simulink model "mrefrobotarm_modified_previous_y_previous_u_previous_ref_pert"  (R2018b)
settings: Solver=FixedStepAuto  StartTime=0.0  StopTime=10  RelTol=1e-3  AbsTol=1e-6
undefined symbols (not defined in the file or in its folder): cc, options
libraries: neural x714, simulink x1
(part 14 of 26)

== system mrefrobotarm_modified_previous_y_previous_u_previous_ref_pert/no_ss_error/Layer 3/LW{3,2} ==
  "ad{3,2}" : Inport  PortDimensions=10
      mask Display: e = 0.06;c1 = [120 230 180]/255;c2 = ([120 230 180]+0)/(256+128);c3 = ([120 230 180]+128)/(256+128);patch([0 1 1 0],[0 0 1 1],c1);patch([0 1 1 1-e 1-e 0+e],[0 0 1 1-e 0+e 0+e],c2);patch([0 0 1 1-e 0+e 0+e],[0 1 1 1-e 1-e 0+e],c3);plot([0 1 1 0 0],[0 0 1 1 0]);
  "IW{3,2}(1,:)'" : Constant  Value=[-1.1742149213841346355735595352598465979099273681640625;-0.36956930765582274300840026626246981322765350341796875;-0.020974811427770558014405111180167295970022678375244140625;-0.1621617407977070934865793105927878059446811676025390625;-1.0555440515423846203901803164626471698284149169921875;0.9397318128967075967494793076184578239917755126953125;1.108386888893071908768206412787549197673797607421875;-1.6860005455705617816164476607809774577617645263671875;0.39441695259544518048500094664632342755794525146484375;0.311368724958305309602479837849386967718601226806640625]
      mask Display: e = 0.06;c1 = [120 150 230]/255;c2 = ([120 150 230]+0)/383;c3 = ([120 150 230]+128)/383;patch([0 1 1 0],[0 0 1 1],c1);patch([0 1 1 1-e 1-e 0+e],[0 0 1 1-e 0+e 0+e],c2);patch([0 0 1 1-e 0+e 0+e],[0 1 1 1-e 1-e 0+e],c3);plot([0 1 1 0 0],[0 0 1 1 0]);disp('weights');
  "IW{3,2}(10,:)'" : Constant  Value=[1.2868963402164153020379444569698534905910491943359375;1.0043335498955787699060238082893192768096923828125;0.357778577002095532488823437233804725110530853271484375;0.125142367753036942712441259573097340762615203857421875;0.329491920370458657441048444525222294032573699951171875;0.3719554364254389344779383463901467621326446533203125;0.094035472804396447177310847109765745699405670166015625;-1.5356693414710511635945522357360459864139556884765625;-0.234492704566690746137425094275386072695255279541015625;0.76033474886525265201697720840456895530223846435546875]
      mask Display: e = 0.06;c1 = [120 150 230]/255;c2 = ([120 150 230]+0)/383;c3 = ([120 150 230]+128)/383;patch([0 1 1 0],[0 0 1 1],c1);patch([0 1 1 1-e 1-e 0+e],[0 0 1 1-e 0+e 0+e],c2);patch([0 0 1 1-e 0+e 0+e],[0 1 1 1-e 1-e 0+e],c3);plot([0 1 1 0 0],[0 0 1 1 0]);disp('weights');
  "IW{3,2}(2,:)'" : Constant  Value=[-0.79821657120366451554360764930606819689273834228515625;-0.3531049846577680728643144902889616787433624267578125;-0.07096205186676474152562832387047819793224334716796875;1.0162264331966504027349174066330306231975555419921875;-0.04359937457296637897119495619335793890058994293212890625;-0.65589298183328781366441262434818781912326812744140625;-1.0034240677702126465220544559997506439685821533203125;-0.178302261212416823799031817543436773121356964111328125;0.26934055472063522795878043325501494109630584716796875;0.7890398483409157837087377629359252750873565673828125]
      mask Display: e = 0.06;c1 = [120 150 230]/255;c2 = ([120 150 230]+0)/383;c3 = ([120 150 230]+128)/383;patch([0 1 1 0],[0 0 1 1],c1);patch([0 1 1 1-e 1-e 0+e],[0 0 1 1-e 0+e 0+e],c2);patch([0 0 1 1-e 0+e 0+e],[0 1 1 1-e 1-e 0+e],c3);plot([0 1 1 0 0],[0 0 1 1 0]);disp('weights');
  "IW{3,2}(3,:)'" : Constant  Value=[0.34998478961192713843075807744753547012805938720703125;0.66241428248508438247910135032725520431995391845703125;0.1149456925372841775701004962684237398207187652587890625;-0.34497320121806829273936045865411870181560516357421875;-1.151869423380677659451976069249212741851806640625;-0.2339138016921568363759575959193171001970767974853515625;-0.494599686326340937103651640427415259182453155517578125;0.149782276593690977239958783684414811432361602783203125;0.30087508159218778747145961460773833096027374267578125;-1.0897169507045614267326527624391019344329833984375]
      mask Display: e = 0.06;c1 = [120 150 230]/255;c2 = ([120 150 230]+0)/383;c3 = ([120 150 230]+128)/383;patch([0 1 1 0],[0 0 1 1],c1);patch([0 1 1 1-e 1-e 0+e],[0 0 1 1-e 0+e 0+e],c2);patch([0 0 1 1-e 0+e 0+e],[0 1 1 1-e 1-e 0+e],c3);plot([0 1 1 0 0],[0 0 1 1 0]);disp('weights');
  "IW{3,2}(4,:)'" : Constant  Value=[-0.06940107506443075890967264740538666956126689910888671875;0.06031549876058779624532490970523213036358356475830078125;-0.258147786648753874150230558370822109282016754150390625;-0.0329451661351574387470719784687389619648456573486328125;0.93910292630476110975479286935296840965747833251953125;0.89089233434477754780544955792720429599285125732421875;-0.560766298108745786521467380225658416748046875;-0.72585852285035645792277136933989822864532470703125;0.674225279114710307482027928926981985569000244140625;0.1249268934935323371870907749325851909816265106201171875]
      mask Display: e = 0.06;c1 = [120 150 230]/255;c2 = ([120 150 230]+0)/383;c3 = ([120 150 230]+128)/383;patch([0 1 1 0],[0 0 1 1],c1);patch([0 1 1 1-e 1-e 0+e],[0 0 1 1-e 0+e 0+e],c2);patch([0 0 1 1-e 0+e 0+e],[0 1 1 1-e 1-e 0+e],c3);plot([0 1 1 0 0],[0 0 1 1 0]);disp('weights');
  "IW{3,2}(5,:)'" : Constant  Value=[1.0319694087142163851922305184416472911834716796875;-0.6356320185586259441379297641105949878692626953125;0.627606968594268010974701610393822193145751953125;-0.60009465064882083762398679027683101594448089599609375;0.36085902571910588587655865921988151967525482177734375;0.0166213576772036956963329856762356939725577831268310546875;0.68217943372506295585111502077779732644557952880859375;-0.260281007332698488543343273704522289335727691650390625;0.4773504187563932799065469225752167403697967529296875;-0.246983657567856285108831571051268838346004486083984375]
      mask Display: e = 0.06;c1 = [120 150 230]/255;c2 = ([120 150 230]+0)/383;c3 = ([120 150 230]+128)/383;patch([0 1 1 0],[0 0 1 1],c1);patch([0 1 1 1-e 1-e 0+e],[0 0 1 1-e 0+e 0+e],c2);patch([0 0 1 1-e 0+e 0+e],[0 1 1 1-e 1-e 0+e],c3);plot([0 1 1 0 0],[0 0 1 1 0]);disp('weights');
  "IW{3,2}(6,:)'" : Constant  Value=[0.59600639630389962153600436067790724337100982666015625;-0.6219517438347332838333159088506363332271575927734375;-0.28957206042188088357391961835674010217189788818359375;-0.6317708261151226967200500439503230154514312744140625;0.7916489865234155320905529151787050068378448486328125;1.1118173714307049149141448651789687573909759521484375;0.95397976829716701896444419617182575166225433349609375;0.264598423771943369597892115052673034369945526123046875;0.36001495974812003364462498211651109158992767333984375;0.43069856328655531374494103147299028933048248291015625]
      mask Display: e = 0.06;c1 = [120 150 230]/255;c2 = ([120 150 230]+0)/383;c3 = ([120 150 230]+128)/383;patch([0 1 1 0],[0 0 1 1],c1);patch([0 1 1 1-e 1-e 0+e],[0 0 1 1-e 0+e 0+e],c2);patch([0 0 1 1-e 0+e 0+e],[0 1 1 1-e 1-e 0+e],c3);plot([0 1 1 0 0],[0 0 1 1 0]);disp('weights');
  "IW{3,2}(7,:)'" : Constant  Value=[0.8347467852459591330926969021675176918506622314453125;0.64027222919503190556866911720135249197483062744140625;0.51949179774282805421847797333612106740474700927734375;0.330143188575668988793410107973613776266574859619140625;1.1088920656695460120744201049092225730419158935546875;-0.85106155681901174414605293350177817046642303466796875;-0.85451872016597718584307585842907428741455078125;-0.459549904446422186055087877321057021617889404296875;0.282431179270222931787515108226216398179531097412109375;-0.37750346721447958220352347780135460197925567626953125]
      mask Display: e = 0.06;c1 = [120 150 230]/255;c2 = ([120 150 230]+0)/383;c3 = ([120 150 230]+128)/383;patch([0 1 1 0],[0 0 1 1],c1);patch([0 1 1 1-e 1-e 0+e],[0 0 1 1-e 0+e 0+e],c2);patch([0 0 1 1-e 0+e 0+e],[0 1 1 1-e 1-e 0+e],c3);plot([0 1 1 0 0],[0 0 1 1 0]);disp('weights');
  "IW{3,2}(8,:)'" : Constant  Value=[0.34325135738398848683772257572854869067668914794921875;-1.01090554861465253821961596258915960788726806640625;1.302095617056524989862964503117837011814117431640625;-1.019798546469042666018367526703514158725738525390625;-1.9669407327809864671763762089540250599384307861328125;0.2982089316163587522368061399902217090129852294921875;0.04332335823831089116620063350637792609632015228271484375;-0.074115637045339133326393721290514804422855377197265625;0.54303975452732922146736882496043108403682708740234375;-0.1028235277364488720053259385167621076107025146484375]
      mask Display: e = 0.06;c1 = [120 150 230]/255;c2 = ([120 150 230]+0)/383;c3 = ([120 150 230]+128)/383;patch([0 1 1 0],[0 0 1 1],c1);patch([0 1 1 1-e 1-e 0+e],[0 0 1 1-e 0+e 0+e],c2);patch([0 0 1 1-e 0+e 0+e],[0 1 1 1-e 1-e 0+e],c3);plot([0 1 1 0 0],[0 0 1 1 0]);disp('weights');
  "IW{3,2}(9,:)'" : Constant  Value=[-0.2519934093643081407520867287530563771724700927734375;0.89673409560586414546179412354831583797931671142578125;-0.3290727524169818618560157119645737111568450927734375;-0.78288240927482222186739591052173636853694915771484375;0.357415489622151583137821262425859458744525909423828125;-0.0396763127742645327344916950096376240253448486328125;0.26571572727522230206176345745916478335857391357421875;0.65064151536380887552724061606568284332752227783203125;-0.2531486350804550422566308043315075337886810302734375;-0.375085198445921974563788126033614389598369598388671875]
      mask Display: e = 0.06;c1 = [120 150 230]/255;c2 = ([120 150 230]+0)/383;c3 = ([120 150 230]+128)/383;patch([0 1 1 0],[0 0 1 1],c1);patch([0 1 1 1-e 1-e 0+e],[0 0 1 1-e 0+e 0+e],c2);patch([0 0 1 1-e 0+e 0+e],[0 1 1 1-e 1-e 0+e],c3);plot([0 1 1 0 0],[0 0 1 1 0]);disp('weights');
  Mux : Mux  Inputs=10
      mask Display: e = 0.06;c1 = [120 150 230]/255;c2 = ([120 150 230]+0)/383;c3 = ([120 150 230]+128)/383;patch([0 1 1 0],[0 0 1 1],c1);patch([0 1 1 1-e 1-e 0+e],[0 0 1 1-e 0+e 0+e],c2);patch([0 0 1 1-e 0+e 0+e],[0 1 1 1-e 1-e 0+e],c3);plot([0 1 1 0 0],[0 0 1 1 0]);disp('Mux');
  dotprod{1..10} (10 alike) : neural/Weight Functions/dotprod
  "lz{3,2}" : Outport
      mask Display: e = 0.06;c1 = [120 230 180]/255;c2 = ([120 230 180]+0)/(256+128);c3 = ([120 230 180]+128)/(256+128);patch([0 1 1 0],[0 0 1 1],c1);patch([0 1 1 1-e 1-e 0+e],[0 0 1 1-e 0+e 0+e],c2);patch([0 0 1 1-e 0+e 0+e],[0 1 1 1-e 1-e 0+e],c3);plot([0 1 1 0 0],[0 0 1 1 0]);
  wires:
  "IW{3,2}(1,:)'"/1 -> dotprod1/1
  "ad{3,2}"/1 -> dotprod1/2, dotprod2/2, dotprod3/2, dotprod4/2, dotprod5/2, dotprod6/2, dotprod7/2, dotprod8/2, dotprod9/2, dotprod10/2
  dotprod1/1 -> Mux/1
  "IW{3,2}(2,:)'"/1 -> dotprod2/1
  dotprod2/1 -> Mux/2
  "IW{3,2}(3,:)'"/1 -> dotprod3/1
  dotprod3/1 -> Mux/3
  "IW{3,2}(4,:)'"/1 -> dotprod4/1
  dotprod4/1 -> Mux/4
  "IW{3,2}(5,:)'"/1 -> dotprod5/1
  dotprod5/1 -> Mux/5
  "IW{3,2}(6,:)'"/1 -> dotprod6/1
  dotprod6/1 -> Mux/6
  "IW{3,2}(7,:)'"/1 -> dotprod7/1
  dotprod7/1 -> Mux/7
  "IW{3,2}(8,:)'"/1 -> dotprod8/1
  dotprod8/1 -> Mux/8
  "IW{3,2}(9,:)'"/1 -> dotprod9/1
  dotprod9/1 -> Mux/9
  "IW{3,2}(10,:)'"/1 -> dotprod10/1
  dotprod10/1 -> Mux/10
  Mux/1 -> "lz{3,2}"/1

== system mrefrobotarm_modified_previous_y_previous_u_previous_ref_pert/no_ss_error/Layer 4/Delays 1 ==
  "p{4}" : Inport  PortDimensions=10
      mask Display: e = 0.06;c1 = [120 230 180]/255;c2 = ([120 230 180]+0)/(256+128);c3 = ([120 230 180]+128)/(256+128);patch([0 1 1 0],[0 0 1 1],c1);patch([0 1 1 1-e 1-e 0+e],[0 0 1 1-e 0+e 0+e],c2);patch([0 0 1 1-e 0+e 0+e],[0 1 1 1-e 1-e 0+e],c3);plot([0 1 1 0 0],[0 0 1 1 0]);
  mux : Mux  Inputs=1
      mask Display: e = 0.06;c1 = [120 150 230]/255;c2 = ([120 150 230]+0)/383;c3 = ([120 150 230]+128)/383;patch([0 1 1 0],[0 0 1 1],c1);patch([0 1 1 1-e 1-e 0+e],[0 0 1 1-e 0+e 0+e],c2);patch([0 0 1 1-e 0+e 0+e],[0 1 1 1-e 1-e 0+e],c3);plot([0 1 1 0 0],[0 0 1 1 0]);disp('Mux')
  "pd{4,3}" : Outport
      mask Display: e = 0.06;c1 = [120 230 180]/255;c2 = ([120 230 180]+0)/(256+128);c3 = ([120 230 180]+128)/(256+128);patch([0 1 1 0],[0 0 1 1],c1);patch([0 1 1 1-e 1-e 0+e],[0 0 1 1-e 0+e 0+e],c2);patch([0 0 1 1-e 0+e 0+e],[0 1 1 1-e 1-e 0+e],c3);plot([0 1 1 0 0],[0 0 1 1 0]);
  wires:
  "p{4}"/1 -> mux/1
  mux/1 -> "pd{4,3}"/1

== system mrefrobotarm_modified_previous_y_previous_u_previous_ref_pert/no_ss_error/Layer 4/LW{4,3} ==
  "ad{4,3}" : Inport  PortDimensions=10
      mask Display: e = 0.06;c1 = [120 230 180]/255;c2 = ([120 230 180]+0)/(256+128);c3 = ([120 230 180]+128)/(256+128);patch([0 1 1 0],[0 0 1 1],c1);patch([0 1 1 1-e 1-e 0+e],[0 0 1 1-e 0+e 0+e],c2);patch([0 0 1 1-e 0+e 0+e],[0 1 1 1-e 1-e 0+e],c3);plot([0 1 1 0 0],[0 0 1 1 0]);
  "IW{4,3}(1,:)'" : Constant  Value=[-0.2284255511763977342098996814456768333911895751953125;0.326359030917801773430397815900505520403385162353515625;0.7413839295182060862288153657573275268077850341796875;-0.359416929133310414368196461509796790778636932373046875;0.359071647237452495904364013767917640507221221923828125;-0.1211637014833257530721510875082458369433879852294921875;0.128617773868923757074611557982279919087886810302734375;-0.890162829817878975546818764996714890003204345703125;0.957733879752896921644378380733542144298553466796875;1.054540145396258399301814279169775545597076416015625]
      mask Display: e = 0.06;c1 = [120 150 230]/255;c2 = ([120 150 230]+0)/383;c3 = ([120 150 230]+128)/383;patch([0 1 1 0],[0 0 1 1],c1);patch([0 1 1 1-e 1-e 0+e],[0 0 1 1-e 0+e 0+e],c2);patch([0 0 1 1-e 0+e 0+e],[0 1 1 1-e 1-e 0+e],c3);plot([0 1 1 0 0],[0 0 1 1 0]);disp('weights');
  Mux : Mux  Inputs=1
      mask Display: e = 0.06;c1 = [120 150 230]/255;c2 = ([120 150 230]+0)/383;c3 = ([120 150 230]+128)/383;patch([0 1 1 0],[0 0 1 1],c1);patch([0 1 1 1-e 1-e 0+e],[0 0 1 1-e 0+e 0+e],c2);patch([0 0 1 1-e 0+e 0+e],[0 1 1 1-e 1-e 0+e],c3);plot([0 1 1 0 0],[0 0 1 1 0]);disp('Mux');
  dotprod1 : neural/Weight Functions/dotprod
  "lz{4,3}" : Outport
      mask Display: e = 0.06;c1 = [120 230 180]/255;c2 = ([120 230 180]+0)/(256+128);c3 = ([120 230 180]+128)/(256+128);patch([0 1 1 0],[0 0 1 1],c1);patch([0 1 1 1-e 1-e 0+e],[0 0 1 1-e 0+e 0+e],c2);patch([0 0 1 1-e 0+e 0+e],[0 1 1 1-e 1-e 0+e],c3);plot([0 1 1 0 0],[0 0 1 1 0]);
  wires:
  "IW{4,3}(1,:)'"/1 -> dotprod1/1
  "ad{4,3}"/1 -> dotprod1/2
  dotprod1/1 -> Mux/1
  Mux/1 -> "lz{4,3}"/1

== system mrefrobotarm_modified_previous_y_previous_u_previous_ref_pert/sd=0.001/Layer 1/Delays 1 ==
  "p{1}" : Inport  PortDimensions=10
      mask Display: e = 0.06;c1 = [120 230 180]/255;c2 = ([120 230 180]+0)/(256+128);c3 = ([120 230 180]+128)/(256+128);patch([0 1 1 0],[0 0 1 1],c1);patch([0 1 1 1-e 1-e 0+e],[0 0 1 1-e 0+e 0+e],c2);patch([0 0 1 1-e 0+e 0+e],[0 1 1 1-e 1-e 0+e],c3);plot([0 1 1 0 0],[0 0 1 1 0]);
  mux : Mux  Inputs=1
      mask Display: e = 0.06;c1 = [120 150 230]/255;c2 = ([120 150 230]+0)/383;c3 = ([120 150 230]+128)/383;patch([0 1 1 0],[0 0 1 1],c1);patch([0 1 1 1-e 1-e 0+e],[0 0 1 1-e 0+e 0+e],c2);patch([0 0 1 1-e 0+e 0+e],[0 1 1 1-e 1-e 0+e],c3);plot([0 1 1 0 0],[0 0 1 1 0]);disp('Mux')
  "pd{1,1}" : Outport
      mask Display: e = 0.06;c1 = [120 230 180]/255;c2 = ([120 230 180]+0)/(256+128);c3 = ([120 230 180]+128)/(256+128);patch([0 1 1 0],[0 0 1 1],c1);patch([0 1 1 1-e 1-e 0+e],[0 0 1 1-e 0+e 0+e],c2);patch([0 0 1 1-e 0+e 0+e],[0 1 1 1-e 1-e 0+e],c3);plot([0 1 1 0 0],[0 0 1 1 0]);
  wires:
  "p{1}"/1 -> mux/1
  mux/1 -> "pd{1,1}"/1

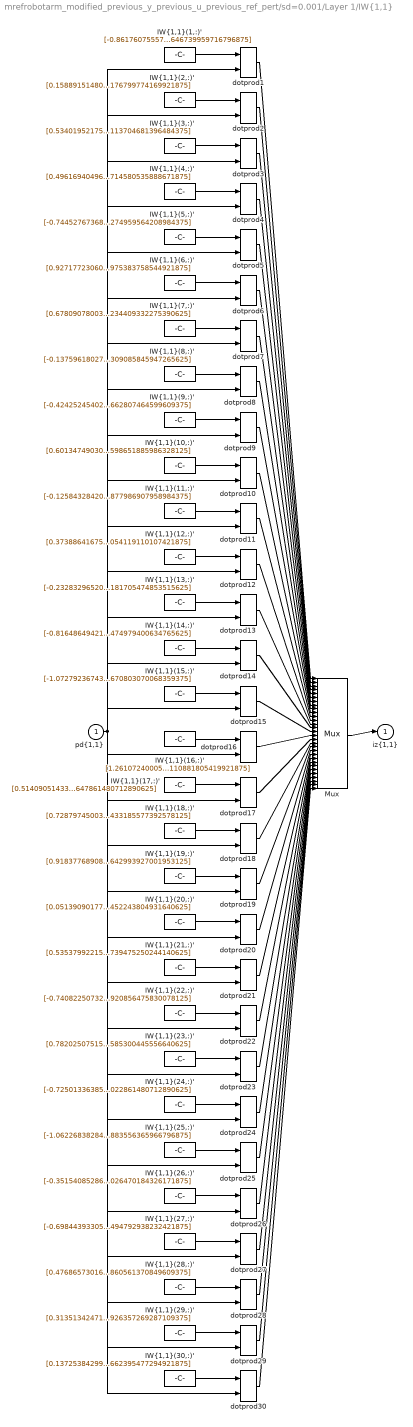
== system mrefrobotarm_modified_previous_y_previous_u_previous_ref_pert/sd=0.001/Layer 1/IW{1,1} ==
  "pd{1,1}" : Inport  PortDimensions=10
      mask Display: e = 0.06;c1 = [120 230 180]/255;c2 = ([120 230 180]+0)/(256+128);c3 = ([120 230 180]+128)/(256+128);patch([0 1 1 0],[0 0 1 1],c1);patch([0 1 1 1-e 1-e 0+e],[0 0 1 1-e 0+e 0+e],c2);patch([0 0 1 1-e 0+e 0+e],[0 1 1 1-e 1-e 0+e],c3);plot([0 1 1 0 0],[0 0 1 1 0]);
  "IW{1,1}(1,:)'" : Constant  Value=[-0.86176075557723141873367467269417829811573028564453125;0.004071028969782842545088730190627757110632956027984619140625;0.9276173767568607342326458820025436580181121826171875;-0.7967440168978880965511280010105110704898834228515625;0.1354921212385334639005662893396220169961452484130859375;0.8229380829797723340135462422040291130542755126953125;-0.89325111752537622589187549237976782023906707763671875;-0.040687801222941966106105837752693332731723785400390625;0.1879890646825829458865797505495720542967319488525390625;0.66378054058433366702018929572659544646739959716796875]
      mask Display: e = 0.06;c1 = [120 150 230]/255;c2 = ([120 150 230]+0)/383;c3 = ([120 150 230]+128)/383;patch([0 1 1 0],[0 0 1 1],c1);patch([0 1 1 1-e 1-e 0+e],[0 0 1 1-e 0+e 0+e],c2);patch([0 0 1 1-e 0+e 0+e],[0 1 1 1-e 1-e 0+e],c3);plot([0 1 1 0 0],[0 0 1 1 0]);disp('Weights');
  "IW{1,1}(10,:)'" : Constant  Value=[0.6013474903013322769851356497383676469326019287109375;0.2357213474255306639992824102591839618980884552001953125;0.0312087080959108920108491247447091154754161834716796875;-0.72882097215190777550475331736379303038120269775390625;0.27025423916619695230423303655697964131832122802734375;-0.15361402603164375779698502810788340866565704345703125;0.78092852510657195796994756165076978504657745361328125;1.1338252142460525373479640620644204318523406982421875;0.8835122077703960741246191901154816150665283203125;-0.57041135401077724953466940860380418598651885986328125]
      mask Display: e = 0.06;c1 = [120 150 230]/255;c2 = ([120 150 230]+0)/383;c3 = ([120 150 230]+128)/383;patch([0 1 1 0],[0 0 1 1],c1);patch([0 1 1 1-e 1-e 0+e],[0 0 1 1-e 0+e 0+e],c2);patch([0 0 1 1-e 0+e 0+e],[0 1 1 1-e 1-e 0+e],c3);plot([0 1 1 0 0],[0 0 1 1 0]);disp('Weights');
  "IW{1,1}(11,:)'" : Constant  Value=[-0.1258432842075885293997572489388403482735157012939453125;-0.95290940317177341700727311035734601318836212158203125;0.3798642085459082995413382377591915428638458251953125;-0.47392543300202205625026863344828598201274871826171875;0.284850629948106226496662429781281389296054840087890625;-0.37713871544512567179907591707888059318065643310546875;0.52725521709343647902556995177292264997959136962890625;0.6632129839156402084654473583213984966278076171875;1.1084132506835449039073182575521059334278106689453125;-0.42571958046212843296274286331026814877986907958984375]
      mask Display: e = 0.06;c1 = [120 150 230]/255;c2 = ([120 150 230]+0)/383;c3 = ([120 150 230]+128)/383;patch([0 1 1 0],[0 0 1 1],c1);patch([0 1 1 1-e 1-e 0+e],[0 0 1 1-e 0+e 0+e],c2);patch([0 0 1 1-e 0+e 0+e],[0 1 1 1-e 1-e 0+e],c3);plot([0 1 1 0 0],[0 0 1 1 0]);disp('Weights');
  "IW{1,1}(12,:)'" : Constant  Value=[0.373886416754146966301419752198853529989719390869140625;-0.53407118968250644197581777916639111936092376708984375;-0.974687317709341360938424259074963629245758056640625;-0.81026545963209606338040202899719588458538055419921875;1.2545756075142449059711680092732422053813934326171875;-1.403611791985415191419406255590729415416717529296875;1.0287428745390150286453945227549411356449127197265625;0.73290349012389544025580789821106009185314178466796875;0.11950116559000185934014126587499049492180347442626953125;-0.6581982943801925056703794325585477054119110107421875]
      mask Display: e = 0.06;c1 = [120 150 230]/255;c2 = ([120 150 230]+0)/383;c3 = ([120 150 230]+128)/383;patch([0 1 1 0],[0 0 1 1],c1);patch([0 1 1 1-e 1-e 0+e],[0 0 1 1-e 0+e 0+e],c2);patch([0 0 1 1-e 0+e 0+e],[0 1 1 1-e 1-e 0+e],c3);plot([0 1 1 0 0],[0 0 1 1 0]);disp('Weights');
  "IW{1,1}(13,:)'" : Constant  Value=[-0.2328329652087623158340790041620493866503238677978515625;0.25214791019473847821785739142796956002712249755859375;-0.857616619290316517520977868116460740566253662109375;0.1597045671382539833160763009800575673580169677734375;-0.89199095776851045069832935041631571948528289794921875;-0.40844745584091957102401693191495724022388458251953125;0.416911726643029556527153545175679028034210205078125;0.44604718664590847776452164907823316752910614013671875;-1.0838179239725198588217836004332639276981353759765625;-1.4845463738733233327593552530743181705474853515625]
      mask Display: e = 0.06;c1 = [120 150 230]/255;c2 = ([120 150 230]+0)/383;c3 = ([120 150 230]+128)/383;patch([0 1 1 0],[0 0 1 1],c1);patch([0 1 1 1-e 1-e 0+e],[0 0 1 1-e 0+e 0+e],c2);patch([0 0 1 1-e 0+e 0+e],[0 1 1 1-e 1-e 0+e],c3);plot([0 1 1 0 0],[0 0 1 1 0]);disp('Weights');
  "IW{1,1}(14,:)'" : Constant  Value=[-0.81648649421498709077837929726229049265384674072265625;-0.1711459426988634902055963493694434873759746551513671875;0.3309884131682216956704678523237816989421844482421875;0.5470694340943669242705027500051073729991912841796875;0.648293249569385832131729330285452306270599365234375;-0.8610077775310236436467903331504203379154205322265625;0.036703737521726009784828193005523644387722015380859375;-0.445491607745406081875216841581277549266815185546875;0.75751953895534140936973699353984557092189788818359375;0.067524437334262776833071484361425973474979400634765625]
      mask Display: e = 0.06;c1 = [120 150 230]/255;c2 = ([120 150 230]+0)/383;c3 = ([120 150 230]+128)/383;patch([0 1 1 0],[0 0 1 1],c1);patch([0 1 1 1-e 1-e 0+e],[0 0 1 1-e 0+e 0+e],c2);patch([0 0 1 1-e 0+e 0+e],[0 1 1 1-e 1-e 0+e],c3);plot([0 1 1 0 0],[0 0 1 1 0]);disp('Weights');
  "IW{1,1}(15,:)'" : Constant  Value=[-1.07279236743805572729115738184191286563873291015625;-0.22077776363054368857774534262716770172119140625;-1.1441750592332462499456369187100790441036224365234375;-0.0243684922136943975246037297210932592861354351043701171875;0.6338152544858817183381916038342751562595367431640625;-0.3991749720177695248679583528428338468074798583984375;-0.033335841958008184671147233757437788881361484527587890625;-0.405257397821079445865422030692570842802524566650390625;0.5599912552127384035571822096244432032108306884765625;-0.91172899721163103148313666679314337670803070068359375]
      mask Display: e = 0.06;c1 = [120 150 230]/255;c2 = ([120 150 230]+0)/383;c3 = ([120 150 230]+128)/383;patch([0 1 1 0],[0 0 1 1],c1);patch([0 1 1 1-e 1-e 0+e],[0 0 1 1-e 0+e 0+e],c2);patch([0 0 1 1-e 0+e 0+e],[0 1 1 1-e 1-e 0+e],c3);plot([0 1 1 0 0],[0 0 1 1 0]);disp('Weights');
  "IW{1,1}(16,:)'" : Constant  Value=[1.261072400056214792840592053835280239582061767578125;-0.448328322608864626719338275506743229925632476806640625;0.2280649357326325343819917179644107818603515625;-0.31922125582217242278915136921568773686885833740234375;2.2790899227644043634199988446198403835296630859375;-0.74094992287071204106752020379644818603992462158203125;-0.06839834232064727348454624689111369661986827850341796875;-0.361411436047278156191708831102005206048488616943359375;-0.274032669218069013794547572615556418895721435546875;0.431462257503983870332575634165550582110881805419921875]
      mask Display: e = 0.06;c1 = [120 150 230]/255;c2 = ([120 150 230]+0)/383;c3 = ([120 150 230]+128)/383;patch([0 1 1 0],[0 0 1 1],c1);patch([0 1 1 1-e 1-e 0+e],[0 0 1 1-e 0+e 0+e],c2);patch([0 0 1 1-e 0+e 0+e],[0 1 1 1-e 1-e 0+e],c3);plot([0 1 1 0 0],[0 0 1 1 0]);disp('Weights');
  "IW{1,1}(17,:)'" : Constant  Value=[0.5140905143300018576013599158613942563533782958984375;-0.9116222129188285006051728487364016473293304443359375;-0.1962638231180134085196442583765019662678241729736328125;0.186268042418468227072736453919787891209125518798828125;-0.1420763900966267867520542722559184767305850982666015625;-0.019898823210212468470814428656012751162052154541015625;-0.650313148725484513335004521650262176990509033203125;-0.8810028290455473864994928590022027492523193359375;-0.41969576868875713149265038737212307751178741455078125;0.9138742157549766265134394416236318647861480712890625]
      mask Display: e = 0.06;c1 = [120 150 230]/255;c2 = ([120 150 230]+0)/383;c3 = ([120 150 230]+128)/383;patch([0 1 1 0],[0 0 1 1],c1);patch([0 1 1 1-e 1-e 0+e],[0 0 1 1-e 0+e 0+e],c2);patch([0 0 1 1-e 0+e 0+e],[0 1 1 1-e 1-e 0+e],c3);plot([0 1 1 0 0],[0 0 1 1 0]);disp('Weights');
  "IW{1,1}(18,:)'" : Constant  Value=[0.728797450031771543166314586414955556392669677734375;-1.1059143967640452377310111842234618961811065673828125;-0.2346485878811759573370210318898898549377918243408203125;-0.2398650213650481977101236452654120512306690216064453125;0.98391225572087848139091192933847196400165557861328125;-0.6467316438353230001467863985453732311725616455078125;0.4068445129430180440266440200502984225749969482421875;0.471891804091633393358762305069831199944019317626953125;0.23388680604045009037150748554267920553684234619140625;-0.46059395380301204614426069383625872433185577392578125]
      mask Display: e = 0.06;c1 = [120 150 230]/255;c2 = ([120 150 230]+0)/383;c3 = ([120 150 230]+128)/383;patch([0 1 1 0],[0 0 1 1],c1);patch([0 1 1 1-e 1-e 0+e],[0 0 1 1-e 0+e 0+e],c2);patch([0 0 1 1-e 0+e 0+e],[0 1 1 1-e 1-e 0+e],c3);plot([0 1 1 0 0],[0 0 1 1 0]);disp('Weights');
  "IW{1,1}(19,:)'" : Constant  Value=[0.91837768908570927006707051987177692353725433349609375;-0.59105909328982153549958411531406454741954803466796875;0.337677288428792798935518248981679789721965789794921875;-0.32801393089185160167886579074547626078128814697265625;-1.476581525623521518042480238364078104496002197265625;1.360454205675157624000348732806742191314697265625;0.1975920020602131843556747980983345769345760345458984375;0.136979522782758766918931314648943953216075897216796875;-0.278310726068780767139543286248226650059223175048828125;0.408523632288254834321605812874622642993927001953125]
      mask Display: e = 0.06;c1 = [120 150 230]/255;c2 = ([120 150 230]+0)/383;c3 = ([120 150 230]+128)/383;patch([0 1 1 0],[0 0 1 1],c1);patch([0 1 1 1-e 1-e 0+e],[0 0 1 1-e 0+e 0+e],c2);patch([0 0 1 1-e 0+e 0+e],[0 1 1 1-e 1-e 0+e],c3);plot([0 1 1 0 0],[0 0 1 1 0]);disp('Weights');
  "IW{1,1}(2,:)'" : Constant  Value=[0.15889151480007679406725173976155929267406463623046875;0.90848432029205439253161102897138334810733795166015625;0.64155091748254111649885089718736708164215087890625;0.56679185884230853798015914435382001101970672607421875;-0.96727157763341597984663167153485119342803955078125;0.144696114956844257282142507392563857138156890869140625;0.15912836727355628152480448989081196486949920654296875;-0.51200285154880742499727830363553948700428009033203125;0.0045477239156999360591981940160621888935565948486328125;1.12206226026558919528497426654212176799774169921875]
      mask Display: e = 0.06;c1 = [120 150 230]/255;c2 = ([120 150 230]+0)/383;c3 = ([120 150 230]+128)/383;patch([0 1 1 0],[0 0 1 1],c1);patch([0 1 1 1-e 1-e 0+e],[0 0 1 1-e 0+e 0+e],c2);patch([0 0 1 1-e 0+e 0+e],[0 1 1 1-e 1-e 0+e],c3);plot([0 1 1 0 0],[0 0 1 1 0]);disp('Weights');
  "IW{1,1}(20,:)'" : Constant  Value=[0.051390901776852758453539848915170296095311641693115234375;-0.47491168190918731095706561973202042281627655029296875;-0.088706260989326934929266599283437244594097137451171875;-0.46533269759354267680606653811992146074771881103515625;1.5224736179922244705409184462041594088077545166015625;0.72387056923248060957831739870016463100910186767578125;0.588027855543530986182076958357356488704681396484375;-0.001544862865131038133503782461275477544404566287994384765625;-0.5252438341891798589955442366772331297397613525390625;-0.232891549258051500093102958999224938452243804931640625]
      mask Display: e = 0.06;c1 = [120 150 230]/255;c2 = ([120 150 230]+0)/383;c3 = ([120 150 230]+128)/383;patch([0 1 1 0],[0 0 1 1],c1);patch([0 1 1 1-e 1-e 0+e],[0 0 1 1-e 0+e 0+e],c2);patch([0 0 1 1-e 0+e 0+e],[0 1 1 1-e 1-e 0+e],c3);plot([0 1 1 0 0],[0 0 1 1 0]);disp('Weights');
  "IW{1,1}(21,:)'" : Constant  Value=[0.53537992215283092267696929411613382399082183837890625;0.1699732380834374778633133473704219795763492584228515625;-0.77372735546563131681097047476214356720447540283203125;0.5554615267418181456804404660942964255809783935546875;-0.51679619336138760132826064364053308963775634765625;-0.14714231735837068892891466020955704152584075927734375;1.2906650515704238824099547855439595878124237060546875;0.495605598113101120105739028076641261577606201171875;-1.023713888121303039469012219342403113842010498046875;-0.401853255365150874300894656698801554739475250244140625]
      mask Display: e = 0.06;c1 = [120 150 230]/255;c2 = ([120 150 230]+0)/383;c3 = ([120 150 230]+128)/383;patch([0 1 1 0],[0 0 1 1],c1);patch([0 1 1 1-e 1-e 0+e],[0 0 1 1-e 0+e 0+e],c2);patch([0 0 1 1-e 0+e 0+e],[0 1 1 1-e 1-e 0+e],c3);plot([0 1 1 0 0],[0 0 1 1 0]);disp('Weights');
  "IW{1,1}(22,:)'" : Constant  Value=[-0.740822507322084877756651621893979609012603759765625;0.36904664134409059794705854073981754481792449951171875;0.57254323597485612395985299372114241123199462890625;-0.511369759229019837931673464481718838214874267578125;-1.48783549169541107204395302687771618366241455078125;0.7858780678826298160544183701858855783939361572265625;0.86056388037199393892251464421860873699188232421875;-0.715690981015516758390049290028400719165802001953125;-0.136678275538785143350395401284913532435894012451171875;-0.89358044855289187058389188678120262920856475830078125]
      mask Display: e = 0.06;c1 = [120 150 230]/255;c2 = ([120 150 230]+0)/383;c3 = ([120 150 230]+128)/383;patch([0 1 1 0],[0 0 1 1],c1);patch([0 1 1 1-e 1-e 0+e],[0 0 1 1-e 0+e 0+e],c2);patch([0 0 1 1-e 0+e 0+e],[0 1 1 1-e 1-e 0+e],c3);plot([0 1 1 0 0],[0 0 1 1 0]);disp('Weights');
  "IW{1,1}(23,:)'" : Constant  Value=[0.78202507515547370342545718813198618590831756591796875;0.25828206134598641341426628059707581996917724609375;-0.2409694427146869266653794738886062987148761749267578125;-0.210082865427679010839057127668638713657855987548828125;-0.81403360514496625466307477836380712687969207763671875;0.74535839689796123952447715055313892662525177001953125;-0.2464559607151478870523675368531257845461368560791015625;0.8493612797300034156222636738675646483898162841796875;-0.56975882470041827598805639354395680129528045654296875;-0.51598667189669955579489624142297543585300445556640625]
      mask Display: e = 0.06;c1 = [120 150 230]/255;c2 = ([120 150 230]+0)/383;c3 = ([120 150 230]+128)/383;patch([0 1 1 0],[0 0 1 1],c1);patch([0 1 1 1-e 1-e 0+e],[0 0 1 1-e 0+e 0+e],c2);patch([0 0 1 1-e 0+e 0+e],[0 1 1 1-e 1-e 0+e],c3);plot([0 1 1 0 0],[0 0 1 1 0]);disp('Weights');
  "IW{1,1}(24,:)'" : Constant  Value=[-0.72501336385004788720465285223326645791530609130859375;-0.55248724362162782153262696738238446414470672607421875;0.29080096265734367566579976482898928225040435791015625;-0.22723773447624584509441092450288124382495880126953125;0.7093191664194573586854630775633268058300018310546875;-0.58886716476370881689916814138996414840221405029296875;-0.49599038221216640298649735996150411665439605712890625;-0.1682957058340164568921437648896244354546070098876953125;-0.6867623859151088527852380138938315212726593017578125;0.94560397275884222612063467749976553022861480712890625]
      mask Display: e = 0.06;c1 = [120 150 230]/255;c2 = ([120 150 230]+0)/383;c3 = ([120 150 230]+128)/383;patch([0 1 1 0],[0 0 1 1],c1);patch([0 1 1 1-e 1-e 0+e],[0 0 1 1-e 0+e 0+e],c2);patch([0 0 1 1-e 0+e 0+e],[0 1 1 1-e 1-e 0+e],c3);plot([0 1 1 0 0],[0 0 1 1 0]);disp('Weights');
  "IW{1,1}(25,:)'" : Constant  Value=[-1.0622683828482750723054550689994357526302337646484375;-0.103486362899913031387910677949548698961734771728515625;-0.31182807265763112791745470531168393790721893310546875;-0.332186788240231456459383707624510861933231353759765625;0.73374329573604846199685880492324940860271453857421875;-0.042661249067794469735925844133817008696496486663818359375;-0.86231787364117506999861006988794542849063873291015625;-0.8329796760272614175590888407896272838115692138671875;0.194720388816659262243291550475987605750560760498046875;0.56859411845522611628211961942724883556365966796875]
      mask Display: e = 0.06;c1 = [120 150 230]/255;c2 = ([120 150 230]+0)/383;c3 = ([120 150 230]+128)/383;patch([0 1 1 0],[0 0 1 1],c1);patch([0 1 1 1-e 1-e 0+e],[0 0 1 1-e 0+e 0+e],c2);patch([0 0 1 1-e 0+e 0+e],[0 1 1 1-e 1-e 0+e],c3);plot([0 1 1 0 0],[0 0 1 1 0]);disp('Weights');
  "IW{1,1}(26,:)'" : Constant  Value=[-0.3515408528609091920458240565494634211063385009765625;-0.363695176945070086649280938217998482286930084228515625;0.63434547018283937713789555346011184155941009521484375;0.136475213055885780111253779978142119944095611572265625;0.6071923157265555204276097356341779232025146484375;-1.6698633602170993572855195452575571835041046142578125;-0.66248865427385761339706959915929473936557769775390625;-0.203884932577403532594217949736048467457294464111328125;-0.375452002578146704081518691964447498321533203125;0.472411031202594144939865827836911194026470184326171875]
      mask Display: e = 0.06;c1 = [120 150 230]/255;c2 = ([120 150 230]+0)/383;c3 = ([120 150 230]+128)/383;patch([0 1 1 0],[0 0 1 1],c1);patch([0 1 1 1-e 1-e 0+e],[0 0 1 1-e 0+e 0+e],c2);patch([0 0 1 1-e 0+e 0+e],[0 1 1 1-e 1-e 0+e],c3);plot([0 1 1 0 0],[0 0 1 1 0]);disp('Weights');
  "IW{1,1}(27,:)'" : Constant  Value=[-0.69844393305554752782171590297366492450237274169921875;-0.00986765958850281156566897067250465624965727329254150390625;0.7625224319765588898434316433849744498729705810546875;0.437004436070655033486076490589766763150691986083984375;0.4826404155059871303734553293907083570957183837890625;-0.758808268895144077959002970601432025432586669921875;0.2400813231889213084091494465610594488680362701416015625;-0.903653660790560753213185307686217129230499267578125;0.67750662053201227141840945478179492056369781494140625;0.71610861006808412820845433088834397494792938232421875]
      mask Display: e = 0.06;c1 = [120 150 230]/255;c2 = ([120 150 230]+0)/383;c3 = ([120 150 230]+128)/383;patch([0 1 1 0],[0 0 1 1],c1);patch([0 1 1 1-e 1-e 0+e],[0 0 1 1-e 0+e 0+e],c2);patch([0 0 1 1-e 0+e 0+e],[0 1 1 1-e 1-e 0+e],c3);plot([0 1 1 0 0],[0 0 1 1 0]);disp('Weights');
  "IW{1,1}(28,:)'" : Constant  Value=[0.4768657301616536781097011044039390981197357177734375;-0.603206361382763400769135841983370482921600341796875;0.87090024152630729492585714979213662445545196533203125;-0.68470001491388188252784630094538442790508270263671875;-1.3304665949868221819230029723257757723331451416015625;0.2913988547407198037575426496914587914943695068359375;-0.10752875919783033697996188493561930954456329345703125;-0.8908944700450744935693592196912504732608795166015625;-0.601088803383282854753133506164886057376861572265625;0.333557089919703064762046551550156436860561370849609375]
      mask Display: e = 0.06;c1 = [120 150 230]/255;c2 = ([120 150 230]+0)/383;c3 = ([120 150 230]+128)/383;patch([0 1 1 0],[0 0 1 1],c1);patch([0 1 1 1-e 1-e 0+e],[0 0 1 1-e 0+e 0+e],c2);patch([0 0 1 1-e 0+e 0+e],[0 1 1 1-e 1-e 0+e],c3);plot([0 1 1 0 0],[0 0 1 1 0]);disp('Weights');
  "IW{1,1}(29,:)'" : Constant  Value=[0.31351342471906751274701719012227840721607208251953125;-1.1991393484386441148359381259069778025150299072265625;-0.68285373943655347517278642044402658939361572265625;-0.25161954479379178284403906218358315527439117431640625;0.380416307209268833577908708321047015488147735595703125;-0.8447720809192758029126935070962645113468170166015625;0.42916756566283631446623303418164141476154327392578125;0.11088260520280952825533660188739304430782794952392578125;0.489719057399391866081117541398270986974239349365234375;-0.6465071601992169458839043727493844926357269287109375]
      mask Display: e = 0.06;c1 = [120 150 230]/255;c2 = ([120 150 230]+0)/383;c3 = ([120 150 230]+128)/383;patch([0 1 1 0],[0 0 1 1],c1);patch([0 1 1 1-e 1-e 0+e],[0 0 1 1-e 0+e 0+e],c2);patch([0 0 1 1-e 0+e 0+e],[0 1 1 1-e 1-e 0+e],c3);plot([0 1 1 0 0],[0 0 1 1 0]);disp('Weights');
  "IW{1,1}(3,:)'" : Constant  Value=[0.53401952175301137248908389665302820503711700439453125;0.8595486259722207034172924977610819041728973388671875;0.5299554195843263482146312526310794055461883544921875;0.418089788997092870470595471488195471465587615966796875;0.82575094577399632544967289504711516201496124267578125;0.408959450086427478421313708167872391641139984130859375;0.766237789850783723721860951627604663372039794921875;-0.08792227880332316447553608895759680308401584625244140625;0.50028850307335537284103565980331040918827056884765625;-0.059811430026277610794149808270958601497113704681396484375]
      mask Display: e = 0.06;c1 = [120 150 230]/255;c2 = ([120 150 230]+0)/383;c3 = ([120 150 230]+128)/383;patch([0 1 1 0],[0 0 1 1],c1);patch([0 1 1 1-e 1-e 0+e],[0 0 1 1-e 0+e 0+e],c2);patch([0 0 1 1-e 0+e 0+e],[0 1 1 1-e 1-e 0+e],c3);plot([0 1 1 0 0],[0 0 1 1 0]);disp('Weights');
  "IW{1,1}(30,:)'" : Constant  Value=[0.1372538429975160567675374068130622617900371551513671875;0.76534685538351221456565554035478271543979644775390625;-0.81733702516169870477824588306248188018798828125;0.08128038756643717055450082398238009773194789886474609375;-0.369334266374815645139761954851564951241016387939453125;0.893252736204813491127652014256455004215240478515625;-0.21523128060089946611554978517233394086360931396484375;0.85950230729412846475412379732006229460239410400390625;-0.08405405790746782457301122803983162157237529754638671875;-0.882416849130727154459918892825953662395477294921875]
      mask Display: e = 0.06;c1 = [120 150 230]/255;c2 = ([120 150 230]+0)/383;c3 = ([120 150 230]+128)/383;patch([0 1 1 0],[0 0 1 1],c1);patch([0 1 1 1-e 1-e 0+e],[0 0 1 1-e 0+e 0+e],c2);patch([0 0 1 1-e 0+e 0+e],[0 1 1 1-e 1-e 0+e],c3);plot([0 1 1 0 0],[0 0 1 1 0]);disp('Weights');
  "IW{1,1}(4,:)'" : Constant  Value=[0.496169404960103366253321155454614199697971343994140625;1.531569761132938634062838900717906653881072998046875;0.25583518188486065181308504179469309747219085693359375;0.179967274834431922858613006610539741814136505126953125;-0.8565978571382706352466129828826524317264556884765625;-0.40904925086059595873422267686692066490650177001953125;-0.85591411845070897168596957271802239120006561279296875;0.53692162655286923556019473835476674139499664306640625;-0.30617474851438875038667219996568746864795684814453125;-0.1847843493027147843132951265943120233714580535888671875]
      mask Display: e = 0.06;c1 = [120 150 230]/255;c2 = ([120 150 230]+0)/383;c3 = ([120 150 230]+128)/383;patch([0 1 1 0],[0 0 1 1],c1);patch([0 1 1 1-e 1-e 0+e],[0 0 1 1-e 0+e 0+e],c2);patch([0 0 1 1-e 0+e 0+e],[0 1 1 1-e 1-e 0+e],c3);plot([0 1 1 0 0],[0 0 1 1 0]);disp('Weights');
  "IW{1,1}(5,:)'" : Constant  Value=[-0.74452767368639960476883743467624299228191375732421875;-0.6832674419714581670604047758388333022594451904296875;0.73117642470174060154164408231736160814762115478515625;-0.376210333881531300281864105272688902914524078369140625;1.1787566608795534417453154674149118363857269287109375;-0.7297807864098455610246674041263759136199951171875;-0.10563571931489601496423347271047532558441162109375;-0.67319420503407101374904186741332523524761199951171875;-0.264351540694907349848818967075203545391559600830078125;0.1664879390517107482505565485553233884274959564208984375]
      mask Display: e = 0.06;c1 = [120 150 230]/255;c2 = ([120 150 230]+0)/383;c3 = ([120 150 230]+128)/383;patch([0 1 1 0],[0 0 1 1],c1);patch([0 1 1 1-e 1-e 0+e],[0 0 1 1-e 0+e 0+e],c2);patch([0 0 1 1-e 0+e 0+e],[0 1 1 1-e 1-e 0+e],c3);plot([0 1 1 0 0],[0 0 1 1 0]);disp('Weights');
  "IW{1,1}(6,:)'" : Constant  Value=[0.92717723060867829332210021675564348697662353515625;0.6271814594219071725689218510524369776248931884765625;-0.198887179138560743485442117162165232002735137939453125;0.51085936332537629223082831231295131146907806396484375;-0.145526299339302445101651528602815233170986175537109375;0.82128076689963147583029012821498326957225799560546875;-0.67785449632898975291794840813963674008846282958984375;-0.370858009807393196322067296932800672948360443115234375;-0.6236590304450426724969247516128234565258026123046875;0.6638113265669296492177409163559786975383758544921875]
      mask Display: e = 0.06;c1 = [120 150 230]/255;c2 = ([120 150 230]+0)/383;c3 = ([120 150 230]+128)/383;patch([0 1 1 0],[0 0 1 1],c1);patch([0 1 1 1-e 1-e 0+e],[0 0 1 1-e 0+e 0+e],c2);patch([0 0 1 1-e 0+e 0+e],[0 1 1 1-e 1-e 0+e],c3);plot([0 1 1 0 0],[0 0 1 1 0]);disp('Weights');
  "IW{1,1}(7,:)'" : Constant  Value=[0.67809078003705869353012758438126184046268463134765625;0.498175591495810532460808417454245500266551971435546875;-0.052718823397995863422327289526947424747049808502197265625;-0.61430570988462485093606346708838827908039093017578125;0.6260482320965918834332342157722450792789459228515625;0.53553763509722995816986212957999669015407562255859375;-0.52026845648438124758428102722973562777042388916015625;-0.0055134134284971735018299199282409972511231899261474609375;-0.83930701912191041369482036316185258328914642333984375;-1.2414559196580479127902663094573654234409332275390625]
      mask Display: e = 0.06;c1 = [120 150 230]/255;c2 = ([120 150 230]+0)/383;c3 = ([120 150 230]+128)/383;patch([0 1 1 0],[0 0 1 1],c1);patch([0 1 1 1-e 1-e 0+e],[0 0 1 1-e 0+e 0+e],c2);patch([0 0 1 1-e 0+e 0+e],[0 1 1 1-e 1-e 0+e],c3);plot([0 1 1 0 0],[0 0 1 1 0]);disp('Weights');
  "IW{1,1}(8,:)'" : Constant  Value=[-0.13759618027295139608412455345387570559978485107421875;0.1267467826767685601385693416887079365551471710205078125;0.65044615316725928888530461335903964936733245849609375;-0.54592959875416158244121334064402617514133453369140625;0.80244301177351962106598648460931144654750823974609375;0.63206122927599650562768829331616871058940887451171875;0.671091102356958568719846880412660539150238037109375;0.61082403194554946157524000227567739784717559814453125;0.2441734964090719051110767168211168609559535980224609375;-0.128037173154035122113469924443052150309085845947265625]
      mask Display: e = 0.06;c1 = [120 150 230]/255;c2 = ([120 150 230]+0)/383;c3 = ([120 150 230]+128)/383;patch([0 1 1 0],[0 0 1 1],c1);patch([0 1 1 1-e 1-e 0+e],[0 0 1 1-e 0+e 0+e],c2);patch([0 0 1 1-e 0+e 0+e],[0 1 1 1-e 1-e 0+e],c3);plot([0 1 1 0 0],[0 0 1 1 0]);disp('Weights');
  "IW{1,1}(9,:)'" : Constant  Value=[-0.424252454028887837633732260655960999429225921630859375;-0.463783421847126842152420067577622830867767333984375;0.88736223638707933947245010131155140697956085205078125;-0.648699893867841215211456074030138552188873291015625;-0.7639090746071885984491700583021156489849090576171875;0.30660626649687949818456900175078772008419036865234375;0.26475337483733241139560732335667125880718231201171875;0.77130677156831684015969585743732750415802001953125;-0.16535503637889370498470498205279000103473663330078125;0.12080907758720103861715955417821533046662807464599609375]
      mask Display: e = 0.06;c1 = [120 150 230]/255;c2 = ([120 150 230]+0)/383;c3 = ([120 150 230]+128)/383;patch([0 1 1 0],[0 0 1 1],c1);patch([0 1 1 1-e 1-e 0+e],[0 0 1 1-e 0+e 0+e],c2);patch([0 0 1 1-e 0+e 0+e],[0 1 1 1-e 1-e 0+e],c3);plot([0 1 1 0 0],[0 0 1 1 0]);disp('Weights');
  Mux : Mux  Inputs=30
      mask Display: e = 0.06;c1 = [120 150 230]/255;c2 = ([120 150 230]+0)/383;c3 = ([120 150 230]+128)/383;patch([0 1 1 0],[0 0 1 1],c1);patch([0 1 1 1-e 1-e 0+e],[0 0 1 1-e 0+e 0+e],c2);patch([0 0 1 1-e 0+e 0+e],[0 1 1 1-e 1-e 0+e],c3);plot([0 1 1 0 0],[0 0 1 1 0]);disp('Mux');
  dotprod{1..30} (30 alike) : neural/Weight Functions/dotprod
  "iz{1,1}" : Outport
      mask Display: e = 0.06;c1 = [120 230 180]/255;c2 = ([120 230 180]+0)/(256+128);c3 = ([120 230 180]+128)/(256+128);patch([0 1 1 0],[0 0 1 1],c1);patch([0 1 1 1-e 1-e 0+e],[0 0 1 1-e 0+e 0+e],c2);patch([0 0 1 1-e 0+e 0+e],[0 1 1 1-e 1-e 0+e],c3);plot([0 1 1 0 0],[0 0 1 1 0]);
  wires:
  "IW{1,1}(1,:)'"/1 -> dotprod1/1
  "pd{1,1}"/1 -> dotprod1/2, dotprod2/2, dotprod3/2, dotprod4/2, dotprod5/2, dotprod6/2, dotprod7/2, dotprod8/2, dotprod9/2, dotprod10/2, dotprod11/2, dotprod12/2, dotprod13/2, dotprod14/2, dotprod15/2, dotprod16/2, dotprod17/2, dotprod18/2, dotprod19/2, dotprod20/2, dotprod21/2, dotprod22/2, dotprod23/2, dotprod24/2, dotprod25/2, dotprod26/2, dotprod27/2, dotprod28/2, dotprod29/2, dotprod30/2
  dotprod1/1 -> Mux/1
  "IW{1,1}(2,:)'"/1 -> dotprod2/1
  dotprod2/1 -> Mux/2
  "IW{1,1}(3,:)'"/1 -> dotprod3/1
  dotprod3/1 -> Mux/3
  "IW{1,1}(4,:)'"/1 -> dotprod4/1
  dotprod4/1 -> Mux/4
  "IW{1,1}(5,:)'"/1 -> dotprod5/1
  dotprod5/1 -> Mux/5
  "IW{1,1}(6,:)'"/1 -> dotprod6/1
  dotprod6/1 -> Mux/6
  "IW{1,1}(7,:)'"/1 -> dotprod7/1
  dotprod7/1 -> Mux/7
  "IW{1,1}(8,:)'"/1 -> dotprod8/1
  dotprod8/1 -> Mux/8
  "IW{1,1}(9,:)'"/1 -> dotprod9/1
  dotprod9/1 -> Mux/9
  "IW{1,1}(10,:)'"/1 -> dotprod10/1
  dotprod10/1 -> Mux/10
  "IW{1,1}(11,:)'"/1 -> dotprod11/1
  dotprod11/1 -> Mux/11
  "IW{1,1}(12,:)'"/1 -> dotprod12/1
  dotprod12/1 -> Mux/12
  "IW{1,1}(13,:)'"/1 -> dotprod13/1
  dotprod13/1 -> Mux/13
  "IW{1,1}(14,:)'"/1 -> dotprod14/1
  dotprod14/1 -> Mux/14
  "IW{1,1}(15,:)'"/1 -> dotprod15/1
  dotprod15/1 -> Mux/15
  "IW{1,1}(16,:)'"/1 -> dotprod16/1
  dotprod16/1 -> Mux/16
  "IW{1,1}(17,:)'"/1 -> dotprod17/1
  dotprod17/1 -> Mux/17
  "IW{1,1}(18,:)'"/1 -> dotprod18/1
  dotprod18/1 -> Mux/18
  "IW{1,1}(19,:)'"/1 -> dotprod19/1
  dotprod19/1 -> Mux/19
  "IW{1,1}(20,:)'"/1 -> dotprod20/1
  dotprod20/1 -> Mux/20
  "IW{1,1}(21,:)'"/1 -> dotprod21/1
  dotprod21/1 -> Mux/21
  "IW{1,1}(22,:)'"/1 -> dotprod22/1
  dotprod22/1 -> Mux/22
  "IW{1,1}(23,:)'"/1 -> dotprod23/1
  dotprod23/1 -> Mux/23
  "IW{1,1}(24,:)'"/1 -> dotprod24/1
  dotprod24/1 -> Mux/24
  "IW{1,1}(25,:)'"/1 -> dotprod25/1
  dotprod25/1 -> Mux/25
  "IW{1,1}(26,:)'"/1 -> dotprod26/1
  dotprod26/1 -> Mux/26
  "IW{1,1}(27,:)'"/1 -> dotprod27/1
  dotprod27/1 -> Mux/27
  "IW{1,1}(28,:)'"/1 -> dotprod28/1
  dotprod28/1 -> Mux/28
  "IW{1,1}(29,:)'"/1 -> dotprod29/1
  dotprod29/1 -> Mux/29
  "IW{1,1}(30,:)'"/1 -> dotprod30/1
  dotprod30/1 -> Mux/30
  Mux/1 -> "iz{1,1}"/1

== system mrefrobotarm_modified_previous_y_previous_u_previous_ref_pert/sd=0.001/Layer 2/Delays 1 ==
  "p{2}" : Inport  PortDimensions=30
      mask Display: e = 0.06;c1 = [120 230 180]/255;c2 = ([120 230 180]+0)/(256+128);c3 = ([120 230 180]+128)/(256+128);patch([0 1 1 0],[0 0 1 1],c1);patch([0 1 1 1-e 1-e 0+e],[0 0 1 1-e 0+e 0+e],c2);patch([0 0 1 1-e 0+e 0+e],[0 1 1 1-e 1-e 0+e],c3);plot([0 1 1 0 0],[0 0 1 1 0]);
  mux : Mux  Inputs=1
      mask Display: e = 0.06;c1 = [120 150 230]/255;c2 = ([120 150 230]+0)/383;c3 = ([120 150 230]+128)/383;patch([0 1 1 0],[0 0 1 1],c1);patch([0 1 1 1-e 1-e 0+e],[0 0 1 1-e 0+e 0+e],c2);patch([0 0 1 1-e 0+e 0+e],[0 1 1 1-e 1-e 0+e],c3);plot([0 1 1 0 0],[0 0 1 1 0]);disp('Mux')
  "pd{2,1}" : Outport
      mask Display: e = 0.06;c1 = [120 230 180]/255;c2 = ([120 230 180]+0)/(256+128);c3 = ([120 230 180]+128)/(256+128);patch([0 1 1 0],[0 0 1 1],c1);patch([0 1 1 1-e 1-e 0+e],[0 0 1 1-e 0+e 0+e],c2);patch([0 0 1 1-e 0+e 0+e],[0 1 1 1-e 1-e 0+e],c3);plot([0 1 1 0 0],[0 0 1 1 0]);
  wires:
  "p{2}"/1 -> mux/1
  mux/1 -> "pd{2,1}"/1
